simulink model "WITH_SOFT_SWITCH"  (R2024b)
settings: Solver=ode15s  StartTime=0.0  StopTime=T_sim  MaxStep=1e-6  RelTol=1e-6
InitFcn:
  | run param_file.m
values from neighbouring files (symbols this model uses):
  param = struct()    [param_file.m]
libraries: fl_lib x49, nesl_utility x34, SimscapeFluids_lib x4, eeDcCurrentController x1, ee_lib x1
(part 2 of 2)

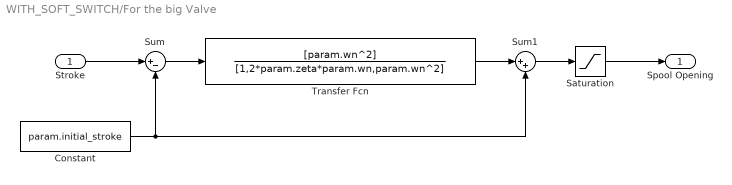
== system WITH_SOFT_SWITCH/For the big Valve ==
  Stroke : Inport
  Constant : Constant  Value=param.initial_stroke
  Saturation : Saturate  UpperLimit=param.stroke  LowerLimit=-param.stroke
  Sum : Sum  Inputs=|+-
  Sum1 : Sum  Inputs=|++
  Transfer Fcn : TransferFcn  Numerator=[param.wn^2]  Denominator=[1,2*param.zeta*param.wn,param.wn^2]
  Spool Opening : Outport
  wires:
  Saturation/1 -> Spool Opening/1
  Sum1/1 -> Saturation/1
  Transfer Fcn/1 -> Sum1/1
  Sum/1 -> Transfer Fcn/1
  Stroke/1 -> Sum/1
  Constant/1 -> Sum1/2, Sum/2

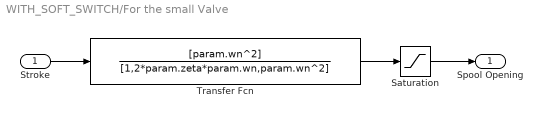
== system WITH_SOFT_SWITCH/For the small Valve ==
  Stroke : Inport
  Saturation : Saturate  UpperLimit=param.stroke  LowerLimit=-param.stroke
  Transfer Fcn : TransferFcn  Numerator=[param.wn^2]  Denominator=[1,2*param.zeta*param.wn,param.wn^2]
  Spool Opening : Outport
  wires:
  Transfer Fcn/1 -> Saturation/1
  Saturation/1 -> Spool Opening/1
  Stroke/1 -> Transfer Fcn/1

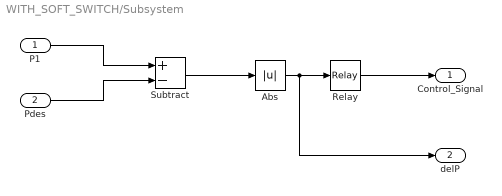
== system WITH_SOFT_SWITCH/Subsystem ==
  P1 : Inport
  Pdes : Inport  Port=2
  Abs : Abs  SaturateOnIntegerOverflow=off
  Relay : Relay  OnSwitchValue=6e5  OffSwitchValue=1e4  OnOutputValue=0  OffOutputValue=1
  Subtract : Sum  Inputs=+-
  Control_Signal : Outport
  delP : Outport  Port=2
  wires:
  P1/1 -> Subtract/1
  Pdes/1 -> Subtract/2
  Subtract/1 -> Abs/1
  Abs/1 -> delP/1, Relay/1
  Relay/1 -> Control_Signal/1

== matlab function WITH_SOFT_SWITCH/Electric Torque Controller1 ==
  data: Kp input; omega input; T_elec output; start_final_velocity input
function T_elec  = fcn(Kp, omega, start_final_velocity)


omega_error = omega -start_final_velocity;

T_elec = - (Kp*omega_error);

== matlab function WITH_SOFT_SWITCH/MATLAB Function5 ==
  data: time input; S_big output; S_small output; param parameter
function [S_big, S_small] = fcn(time, param)


between_switches = param.between_switches;
avoid_bypass_time = param.big_delay;
regen_time = param.regen_time;

first_time = between_switches/2; % At a certain pressure time
second_time = first_time + avoid_bypass_time; % Soft-switch valve advance 
third_time = second_time + regen_time; % Time before switching to middle position
fourth_time = third_time + between_switches; % Time between switches I guess (At a certain pressure)
fifth_time = fourth_time + avoid_bypass_time; 
sixth_time = fifth_time + regen_time;
final_time = sixth_time + between_switches/2;


% The chamber is at a certain pressure
if time < first_time
    S_small = 0;
    S_big = -param.stroke;

% Putting the soft-switch valve in position ahead of time to avoid bypass
elseif time >= first_time && time < second_time
    S_small = param.stroke;
    S_big = -param.stroke;

% Finally changing the pressure or the big valve
% The third_time here is quite important as that defines when the kinetic energy will be conserved.
elseif time >= second_time && time < third_time
    S_small = param.stroke;
    S_big = param.stroke;

% Keeping the soft-switch valve in the middle position, meaning the switching is complete
elseif time >= third_time && time < fourth_time
    S_small = 0;
    S_big = param.stroke;

% Putting the soft-switch valve in position ahead of time to avoid bypass
elseif time >= fourth_time && time < fifth_time
    S_small = -param.stroke;
    S_big = param.stroke;
    
% Finally changing the pressure or the big valve
% The third_time here is quite important as that defines when the kinetic energy will be conserved.
elseif time >= fifth_time && time < sixth_time
    S_small = -param.stroke;
    S_big = -param.stroke;

% Keeping the soft-switch valve in the middle position, meaning the switching is complete
elseif time >= sixth_time && time < final_time
    S_small = 0;
    S_big = -param.stroke;

else
    S_small = 0;
    S_big = -param.stroke;
end

== matlab function WITH_SOFT_SWITCH/MATLAB Function2 ==
  data: Pdes input; S_big output; S_small output; param parameter; Control_signal input
function [S_big, S_small] = fcn(Pdes, param, Control_signal)

if Pdes == param.P_H && Control_signal == 0
    S_big = param.stroke;
    S_small = param.stroke;

elseif Pdes == param.P_M && Control_signal == 0
    S_big = -param.stroke;
    S_small = -param.stroke;

elseif Pdes == param.P_H && Control_signal > 0
    S_big = param.stroke;
    S_small = 0;

elseif Pdes == param.P_M && Control_signal > 0
    S_big = -param.stroke;
    S_small = 0;
    
else
    S_big = 0;
    S_small = 0;
end

== matlab function WITH_SOFT_SWITCH/MATLAB Function3 ==
  data: Power_loss_2 output; P_A_small input; P_B_small input; P_P_small input; P_T_small input; S_small input; Q_A_big input; Qout input; Q_P_small input; Q_T_small input; Power_loss_middle output
function [Power_loss_2, Power_loss_middle] = fcn(P_A_small, P_B_small, P_P_small, P_T_small, S_small, Q_A_big, Qout, Q_P_small, Q_T_small)

Power_loss_middle = (S_small>=-2.5e-3 && S_small<=2.5e-3)*((P_A_small-P_P_small)*Q_P_small + (P_T_small-P_B_small)*Q_P_small + (P_A_small-P_T_small)*Q_T_small + (P_P_small-P_B_small)*Q_T_small);


Power_loss_2 = (S_small>2.5e-3)*((P_A_small-P_P_small)*Q_A_big + (P_T_small-P_B_small)*Qout) ...
              +(S_small<-2.5e-3)*((P_A_small-P_T_small)*Q_A_big + (P_P_small-P_B_small)*Qout)...
              + Power_loss_middle;

== matlab function WITH_SOFT_SWITCH/MATLAB Function6 ==
  data: T_elec_2 input; Elec_Power output; omega input; param parameter; V_elec output; I_elec output
function [Elec_Power, V_elec, I_elec] = fcn(T_elec_2, omega, param)

I_elec = (T_elec_2*omega>0)*(T_elec_2/param.Kt)/param.elec_eff + ...
(T_elec_2*omega<0)*(T_elec_2/param.Kt)*param.elec_eff;

V_elec = (T_elec_2*omega>0)*(omega/param.Kv)/param.elec_eff + ...
    (T_elec_2*omega<0)*(omega/param.Kv)*param.elec_eff;

% Motoring

Elec_Power = I_elec*V_elec;

== matlab function WITH_SOFT_SWITCH/MATLAB Function4 ==
  data: P_H_rail input; P_M_rail input; Q_P_big input; Q_T_big input; Power_out_1 output; Power_out_2 output
function [Power_out_1, Power_out_2] = fcn(P_H_rail, P_M_rail, Q_P_big, Q_T_big)

Power_out_1 = (Q_P_big)*(P_H_rail);

Power_out_2 = (Q_T_big)*(P_M_rail);

== matlab function WITH_SOFT_SWITCH/MATLAB Function1 ==
  data: P1 input; Qout input; Power_out output; param parameter
function Power_out = fcn(P1, Qout, param)

% gamma = 1.4; % Adiabatic process
% Pt = param.P_T;
% 
% Pg = P1-Pt;   % Gauge pressure
% r = P1/Pt;    % Pressure ratio
% e = exp(Pg/param.beta);
% rv = (1/e+param.air*r^(-1/gamma))/(1+param.air);      %Volume ratio
% 
% El=param.beta*(e-(1+Pg/param.beta))+Pt*(e-1);           %Energy in liquid
% Eg=P1/(gamma-1).*(1-r.^(1/gamma-1));          %Energy in gas
% E=(El./e+param.air*Eg.*r.^(-1/gamma))./(1./e+param.air*r.^(-1/gamma));    %Energy in mixture
% W = E-(1./rv-1)*Pt;  %Compressibility (volumetric) energy density
% 
% Power_out = (Qout)*(W+Pg);

Power_out = P1*Qout;
